simulink library "RflySimModelLab"  (R2022a)
settings: Solver=VariableStepAuto  StartTime=0.0  StopTime=10.0  RelTol=1e-3
values from neighbouring files (symbols this model uses):
  ESC = [ESC,ESCTmp]    [USV_init.m]
  motor = [motor,motorTmp]    [USV_init.m]
undefined symbols (not defined in the file or in its folder): LiftDrag
libraries: $bdroot x24, vrlib x3, aerolibasang x1, aerolibtransform2 x1
settings Model: Creator=dream  LastModifiedBy=dzl20201126
settings SolverCC: AlgebraicLoopSolver=TrustRegion
settings DataIOCC: ReturnWorkspaceOutputs=off
settings DebuggingCC: UnconnectedInputMsg=warning  UnconnectedOutputMsg=warning  UnconnectedLineMsg=warning  SFMachineParentedDataDiag=warning  ArithmeticOperatorsInVariantConditions=warning
settings SFSimCC: SimUseLocalCustomCode=off  CustomCodeUndefinedFunction=UseInterfaceOnly
settings RTWCC: RTWUseLocalCustomCode=off

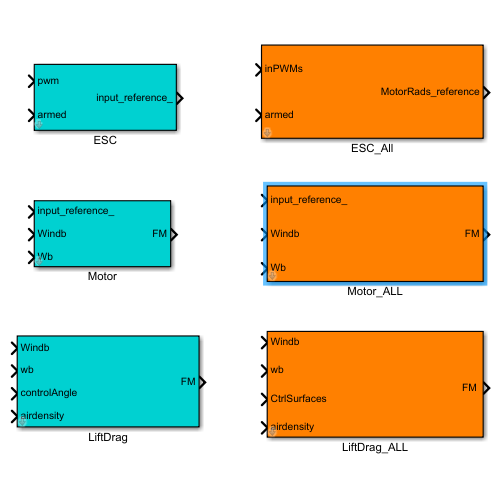
[thumbnail: Simulink's stored preview of the top-level diagram]
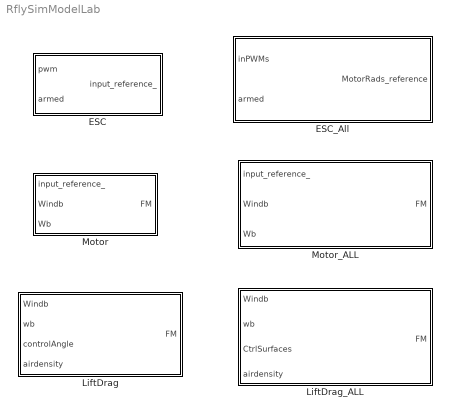
== system RflySimModelLab ==
  ESC : Subsystem  mask{MotorPara=ESC(1)}
      mask prompts: MotorPara "电机名"
  ESC_All : Subsystem  mask{ESCParam=ESC}
      mask prompts: ESCParam "电调参数"
  LiftDrag : Subsystem  mask{LiftDragParam=LiftDrag(1)}
      mask prompts: LiftDragParam "参数结构体"
  LiftDrag_ALL : Subsystem  mask{LiftDrag=LiftDrag}
      mask prompts: LiftDrag "部件参数结构体向量"
  Motor : Subsystem  mask{MotorPara=motor(1)}
      mask prompts: MotorPara "电机名"
  Motor_ALL : Subsystem  mask{MotorParam=motor}
      mask prompts: MotorParam "电机参数"

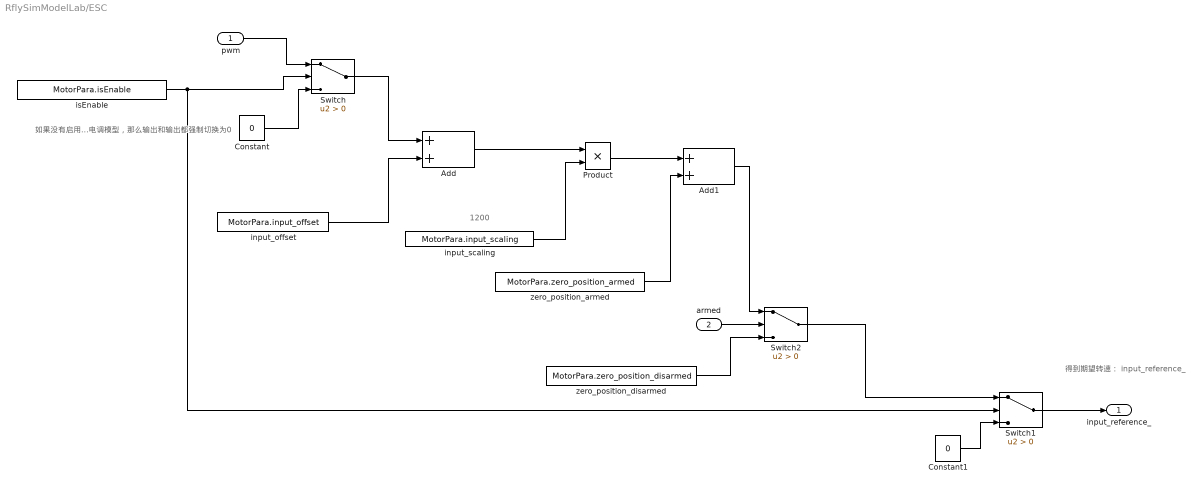
== system RflySimModelLab/ESC ==
  note: 如果没有启用电调模型，那么输出和输出都强制切换为0
  note: 1200
  note: 得到期望转速：
      | input_reference_
  pwm : Inport
  armed : Inport  Port=2
  Add : Sum
  Add1 : Sum
  Constant : Constant  Value=0
  Constant1 : Constant  Value=0
  Product : Product
  Switch : Switch  Criteria=u2 > Threshold  SaturateOnIntegerOverflow=off  InputSameDT=off
  Switch1 : Switch  Criteria=u2 > Threshold  SaturateOnIntegerOverflow=off  InputSameDT=off
  Switch2 : Switch  Criteria=u2 > Threshold  SaturateOnIntegerOverflow=off  InputSameDT=off
  input_offset : Constant  Value=MotorPara.input_offset
  input_scaling : Constant  Value=MotorPara.input_scaling
  isEnable : Constant  Value=MotorPara.isEnable
  zero_position_armed : Constant  Value=MotorPara.zero_position_armed
  zero_position_disarmed : Constant  Value=MotorPara.zero_position_disarmed
  input_reference_ : Outport  VectorParamsAs1DForOutWhenUnconnected=off
  wires:
  Product/1 -> Add1/1
  input_scaling/1 -> Product/2
  pwm/1 -> Switch/1
  Switch2/1 -> Switch1/1
  zero_position_armed/1 -> Add1/2
  input_offset/1 -> Add/2
  Add/1 -> Product/1
  isEnable/1 -> Switch/2, Switch1/2
  Constant/1 -> Switch/3
  Switch/1 -> Add/1
  Constant1/1 -> Switch1/3
  Switch1/1 -> input_reference_/1
  armed/1 -> Switch2/2
  Add1/1 -> Switch2/1
  zero_position_disarmed/1 -> Switch2/3

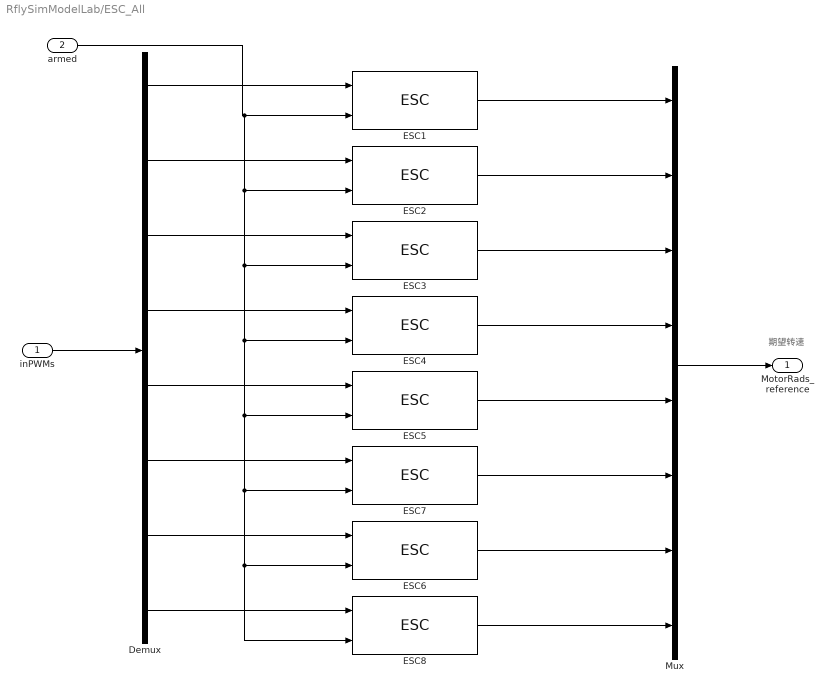
== system RflySimModelLab/ESC_All ==
  note: 期望转速
  inPWMs : Inport  PortDimensions=8
  armed : Inport  Port=2  PortDimensions=1
  Demux : Demux  Outputs=8
  ESC1 : $bdroot/ESC  MotorPara=ESCParam(1)
  ESC2 : $bdroot/ESC  MotorPara=ESCParam(2)
  ESC3 : $bdroot/ESC  MotorPara=ESCParam(3)
  ESC4 : $bdroot/ESC  MotorPara=ESCParam(4)
  ESC5 : $bdroot/ESC  MotorPara=ESCParam(5)
  ESC6 : $bdroot/ESC  MotorPara=ESCParam(7)
  ESC7 : $bdroot/ESC  MotorPara=ESCParam(6)
  ESC8 : $bdroot/ESC  MotorPara=ESCParam(8)
  Mux : Mux  Inputs=8
  MotorRads_reference : Outport  VectorParamsAs1DForOutWhenUnconnected=off
  wires:
  ESC2/1 -> Mux/2
  ESC1/1 -> Mux/1
  Demux/2 -> ESC2/1
  Demux/1 -> ESC1/1
  Demux/3 -> ESC3/1
  ESC3/1 -> Mux/3
  Demux/4 -> ESC4/1
  ESC4/1 -> Mux/4
  Demux/5 -> ESC5/1
  ESC5/1 -> Mux/5
  Demux/6 -> ESC7/1
  ESC7/1 -> Mux/6
  Demux/7 -> ESC6/1
  ESC6/1 -> Mux/7
  Demux/8 -> ESC8/1
  ESC8/1 -> Mux/8
  Mux/1 -> MotorRads_reference/1
  inPWMs/1 -> Demux/1
  armed/1 -> ESC8/2, ESC6/2, ESC7/2, ESC5/2, ESC4/2, ESC3/2, ESC2/2, ESC1/2

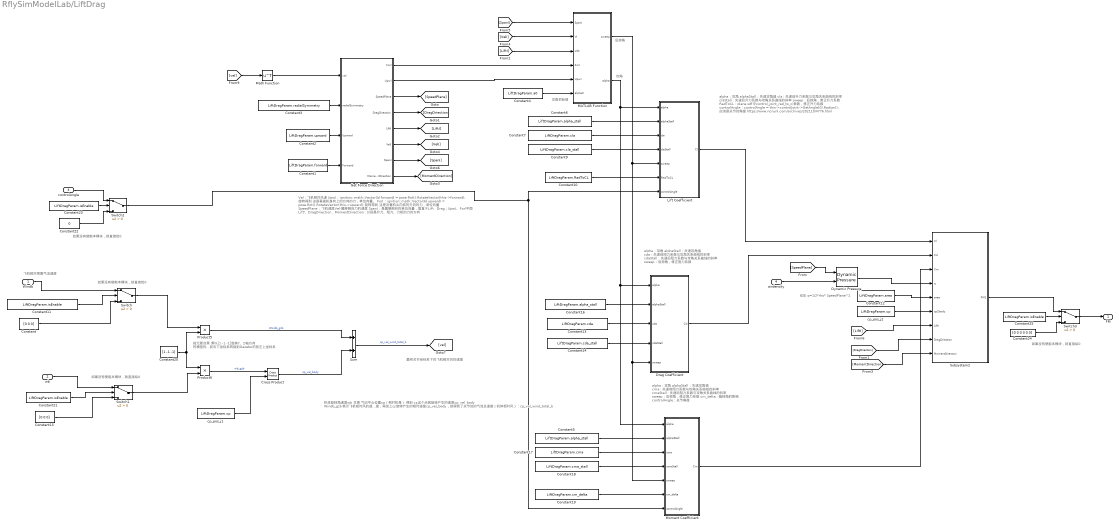
== system RflySimModelLab/LiftDrag ==
  note: alpha：攻角
      | alphaStall：失速攻角值
      | cla：失速前升力系数与攻角关系曲线的斜率
      | claStall：失速后升力系数与攻角关系曲线的斜率
      | sweep：后掠角，修正升力系数
      | RadToCL：plane sdf中control_joint_rad_to_cl参数，修正升力系数
      | controlAngle：controlAngle = this->controlJoint->GetAngle(0).Radian();
      | 应该是关节的角度
      |
      | https://www.ncnynl.com/archives/202110/4776.html
  note: 动压 q=1/2*rho* SpeedPlane^2
  note: 按元素点乘
      | 乘以[1 -1 -1]变换Y、Z轴方向
      | 将模型的前右下坐标系转换到Gazebo的前左上坐标系
  note: 攻角初始值
  note: 机体旋转角速度wb 叉乘 气动中心位置cp（相对机身） 得到 cp这个点因旋转产生的速度cp_vel_body
      |
      | Windb_gzb表示飞机相对风的速度，再加上cp旋转产生的相对速度cp_vel_body，就得到了关节处的气流总速度（机体相对风）：cp_vel_wind_total_b
  note: 如果没有使能本模块，就直接给0
  note: 飞机相对周围气流速度
  note: alpha：攻角
      | alphaStall：失速攻角值
      | cma：失速前阻力系数与攻角关系曲线的斜率
      | cmaStall：失速后阻力系数与攻角关系曲线的斜率
      | sweep：后掠角，修正阻力系数
      | cm_delta：偏转角的影响
      | controlAngle：关节角度
  note: 如果没有使能本模块，就直接给0
  note: 攻角
  note: 如果没有使能本模块，就直接给0
  note: 后掠角
  note: 如果没有使能本模块，就直接给0
  note: 最终关节坐标系下的飞机相对风的速度
  note: Vel：飞机相对风速
      | UpwI：ignition::math::Vector3d forwardI = pose.Rot().RotateVector(this->forward); 旋转得到
      | 	    这是垂直机身向上的方向的力，单位向量。
      | ForI：ignition::math::Vector3d upwardI = pose.Rot().RotateVector(this->upward);旋转得到
      | 	    这是沿着机头向前的方向的力，单位向量
      |
      | SpeedPlane：飞机速度Vel-翼展侧向力的速度
      | SpanI：是翼展侧向的单位向量，垂直于Lift、Drag；UpwI、ForI平面
      | LiftI、DragDriection、MomentDirection：分别是升力、阻力、力矩的力的方向
  note: alpha：攻角
      | alphaStall：失速攻角值
      | cda：失速前阻力系数与攻角关系曲线的斜率
      | cdaStall：失速后阻力系数与攻角关系曲线的斜率
      | sweep：后掠角，修正阻力系数
  Windb : Inport
  wb : Inport  Port=2
  controlAngle : Inport  Port=3
  airdensity : Inport  Port=4
  Constant : Constant  Value=[0 0 0]  VectorParams1D=off
  Constant1 : Constant  Value=LiftDragParam.forward  VectorParams1D=off
  Constant10 : Constant  Value=LiftDragParam.RadToCL
  Constant{11,21,23,25} (4 alike) : Constant  Value=LiftDragParam.isEnable
  Constant12 : Constant  Value=LiftDragParam.area
  Constant13 : Constant  Value=LiftDragParam.cda
  Constant14 : Constant  Value=LiftDragParam.cda_stall
  Constant15 : Constant  Value=[0 0 0]  VectorParams1D=off
  Constant16 : Constant  Value=LiftDragParam.alpha_stall
  Constant17 : Constant  Value=LiftDragParam.cma
  Constant18 : Constant  Value=LiftDragParam.cma_stall
  Constant19 : Constant  Value=LiftDragParam.cm_delta
  Constant2 : Constant  Value=LiftDragParam.upward  VectorParams1D=off
  Constant20 : Constant  Value=[1 -1 -1]  VectorParams1D=off
  Constant22 : Constant  Value=0
  Constant24 : Constant  Value=[0 0 0 0 0 0]
  Constant3 : Constant  Value=LiftDragParam.radialSymmetry
  Constant4 : Constant  Value=LiftDragParam.a0
  Constant5 : Constant  Value=LiftDragParam.alpha_stall
  Constant6 : Constant  Value=LiftDragParam.alpha_stall
  Constant7 : Constant  Value=LiftDragParam.cla
  Constant9 : Constant  Value=LiftDragParam.cla_stall
  Cross Product : vrlib/Utilities/Cross Product
  Drag Coefficient : MATLAB Function  TreatAsAtomicUnit=on
  Dynamic Pressure : aerolibasang/Dynamic Pressure
  Get Force Direction : MATLAB Function  Description=dddddd  TreatAsAtomicUnit=on
  Lift Coefficient : MATLAB Function  TreatAsAtomicUnit=on
  MATLAB Function : MATLAB Function  TreatAsAtomicUnit=on
  Math Function : Math  Operator=transpose  SignedPower=on
  Moment Coefficient : MATLAB Function  TreatAsAtomicUnit=on
  Product5 : Product
  Product6 : Product
  Subsystem2 : Subsystem
  Sum : Sum
  Switch{,1..3} (4 alike) : Switch  Criteria=u2 > Threshold  SaturateOnIntegerOverflow=off  InputSameDT=off
  cp_pos_j1 : Constant  Value=LiftDragParam.cp
  cp_pos_j2 : Constant  Value=LiftDragParam.cp
  FM : Outport  VectorParamsAs1DForOutWhenUnconnected=off
  wires:
  Constant16/1 -> Drag Coefficient/2(alphaStall)
  Windb/1 -> Switch/1
  Sum/1 -> [vel]  "cp_vel_wind_total_b"
  Constant17/1 -> Moment Coefficient/3(cma)
  Constant7/1 -> Lift Coefficient/3(cla)
  Get Force Direction/3(SpeedPlane) -> [SpeedPlane]
  Get Force Direction/6(VelI) -> [VelI]
  Constant19/1 -> Moment Coefficient/6(cm_delta)
  Dynamic Pressure/1 -> Subsystem2/4(q)
  Get Force Direction/7(SpanI) -> [SpanI]
  Constant6/1 -> Lift Coefficient/2(alphaStall)
  Constant13/1 -> Drag Coefficient/3(cda)
  Constant14/1 -> Drag Coefficient/4(cdaStall)
  Constant9/1 -> Lift Coefficient/4(claStall)
  Constant20/1 -> Product5/2, Product6/1
  Constant1/1 -> Get Force Direction/4(Forward)
  [VelI] -> MATLAB Function/2(VI)
  MATLAB Function/1(sweep) -> Lift Coefficient/5(sweep), Drag Coefficient/5(sweep), Moment Coefficient/5(sweep)
  airdensity/1 -> Dynamic Pressure/2
  MATLAB Function/2(alpha) -> Drag Coefficient/1(alpha), Moment Coefficient/1(alpha), Lift Coefficient/1(alpha)
  Get Force Direction/4(DragDirection) -> [DragDriection]
  Constant3/1 -> Get Force Direction/2(radialSymmetry)
  cp_pos_j1/1 -> Cross Product/2
  Constant10/1 -> Lift Coefficient/6(RadToCL)
  Get Force Direction/5(LiftI) -> [LiftI]
  Constant25/1 -> Switch3/2
  Constant5/1 -> Moment Coefficient/2(alphaStall)
  [SpeedPlane] -> Dynamic Pressure/1
  Lift Coefficient/1(Cl) -> Subsystem2/1(Cl)
  Constant4/1 -> MATLAB Function/6(alpha0)
  Moment Coefficient/1(Cm) -> Subsystem2/3(Cm)
  [LiftI] -> Subsystem2/7(LiftI)
  [vel] -> Math Function/1
  cp_pos_j2/1 -> Subsystem2/6(cp2body)
  Cross Product/1 -> Sum/2  "cp_vel_body"
  Get Force Direction/2(UpwI) -> MATLAB Function/5(UpwI)
  [SpanI] -> MATLAB Function/1(SpanI)
  controlAngle/1 -> Switch2/1
  Switch/1 -> Product5/1
  Constant18/1 -> Moment Coefficient/4(cmaStall)
  Get Force Direction/1(ForI) -> MATLAB Function/4(ForI)
  Constant11/1 -> Switch/2
  Get Force Direction/8(MomentDirection) -> [MomentDirection]
  Switch1/1 -> Product6/2
  Product5/1 -> Sum/1  "Windb_gzb"
  Switch2/1 -> Lift Coefficient/7(controlAngle), Moment Coefficient/7(controlAngle)
  Product6/1 -> Cross Product/1  "wb_gzb"
  Constant/1 -> Switch/3
  [MomentDirection] -> Subsystem2/9(MomentDirection)
  Drag Coefficient/1(Cd) -> Subsystem2/2(Cd)
  [DragDriection] -> Subsystem2/8(DragDriection)
  Constant12/1 -> Subsystem2/5(area)
  Constant23/1 -> Switch2/2
  Constant2/1 -> Get Force Direction/3(Upward)
  Subsystem2/1(FM1) -> Switch3/1
  [LiftI] -> MATLAB Function/3(LiftI)
  Constant15/1 -> Switch1/3
  Constant21/1 -> Switch1/2
  Switch3/1 -> FM/1
  wb/1 -> Switch1/1
  Constant24/1 -> Switch3/3
  Math Function/1 -> Get Force Direction/1(vel)
  Constant22/1 -> Switch2/3

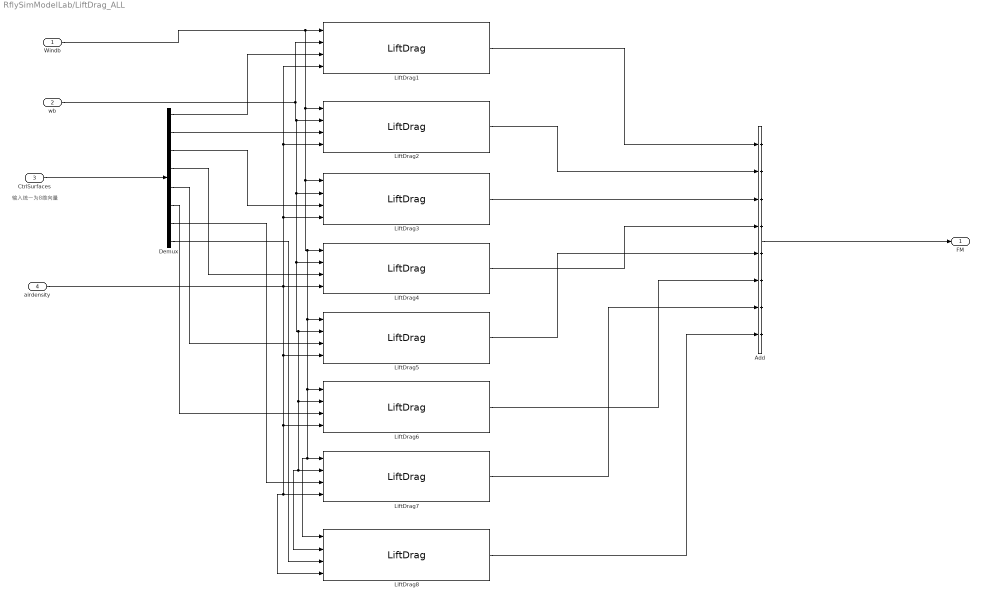
== system RflySimModelLab/LiftDrag_ALL ==
  note: 输入统一为8维向量
  Windb : Inport
  wb : Inport  Port=2
  CtrlSurfaces : Inport  Port=3  PortDimensions=8
  airdensity : Inport  Port=4
  Add : Sum  Inputs=++++++++
  Demux : Demux  Outputs=8
  LiftDrag1 : $bdroot/LiftDrag  LiftDragParam=LiftDrag(1)
  LiftDrag2 : $bdroot/LiftDrag  LiftDragParam=LiftDrag(2)
  LiftDrag3 : $bdroot/LiftDrag  LiftDragParam=LiftDrag(3)
  LiftDrag4 : $bdroot/LiftDrag  LiftDragParam=LiftDrag(4)
  LiftDrag5 : $bdroot/LiftDrag  LiftDragParam=LiftDrag(5)
  LiftDrag6 : $bdroot/LiftDrag  LiftDragParam=LiftDrag(6)
  LiftDrag7 : $bdroot/LiftDrag  LiftDragParam=LiftDrag(7)
  LiftDrag8 : $bdroot/LiftDrag  LiftDragParam=LiftDrag(8)
  "FM " : Outport
  wires:
  Windb/1 -> LiftDrag1/1, LiftDrag2/1, LiftDrag3/1, LiftDrag4/1, LiftDrag5/1, LiftDrag6/1, LiftDrag8/1, LiftDrag7/1
  wb/1 -> LiftDrag1/2, LiftDrag2/2, LiftDrag3/2, LiftDrag4/2, LiftDrag5/2, LiftDrag6/2, LiftDrag8/2, LiftDrag7/2
  Demux/2 -> LiftDrag2/3
  LiftDrag6/1 -> Add/6
  LiftDrag3/1 -> Add/3
  Demux/3 -> LiftDrag3/3
  Demux/4 -> LiftDrag4/3
  LiftDrag5/1 -> Add/5
  Demux/7 -> LiftDrag7/3
  Demux/5 -> LiftDrag5/3
  Demux/1 -> LiftDrag1/3
  airdensity/1 -> LiftDrag3/4, LiftDrag2/4, LiftDrag1/4, LiftDrag4/4, LiftDrag5/4, LiftDrag6/4, LiftDrag8/4, LiftDrag7/4
  Demux/6 -> LiftDrag6/3
  LiftDrag7/1 -> Add/7
  CtrlSurfaces/1 -> Demux/1
  Add/1 -> "FM "/1
  LiftDrag8/1 -> Add/8
  Demux/8 -> LiftDrag8/3
  LiftDrag2/1 -> Add/2
  LiftDrag4/1 -> Add/4
  LiftDrag1/1 -> Add/1

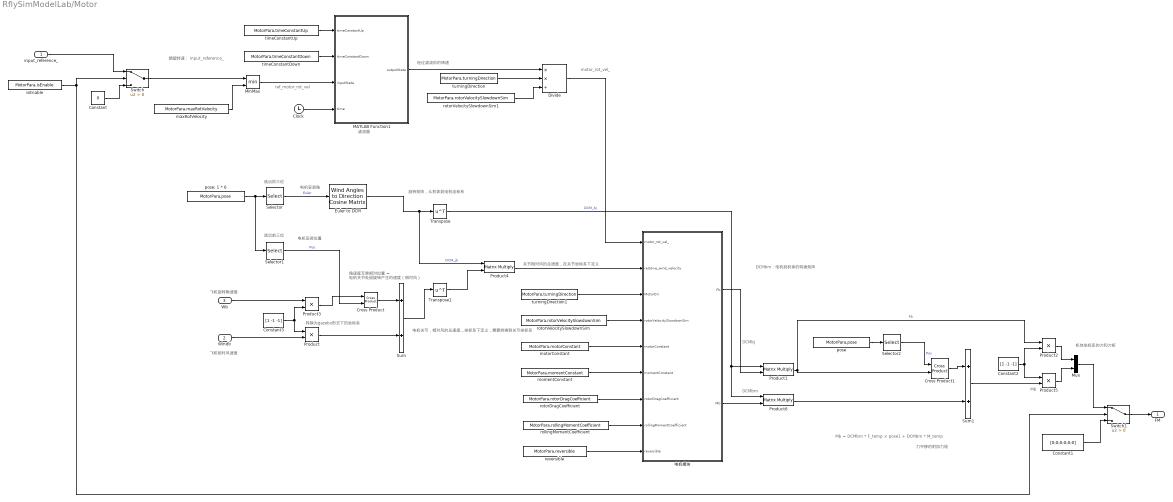
== system RflySimModelLab/Motor ==
  note: 关节相对风的总速度，在关节坐标系下定义
  note: 电机关节，相对风的总速度，在机体坐标系下定义，需要转换到关节坐标系
  note: 角速度叉乘相对位置 = 电机关节处因旋转产生的速度（相对风）
  note: 飞机旋转角速度
  note: 飞机相对风速度
  note: 电机安装位置
  note: 电机安装角
  note: 旋转矩阵，从机体到电机坐标系
  note: 选出后三位
  note: motor_rot_vel_
  note: 转换为gazebo形式下的坐标系
  note: 机体坐标系的力和力矩
  note: 力平移的附加力矩
  note: Mb
  note: DCMbm
  note: DCMbm：电机到机体的转换矩阵
  note: Mb = DCMbm * F_temp × pose1 + DCMbm * M_temp
  note: DCMbj
  note: ref_motor_rot_vel
  note: 经过滤波后的转速
  note: 滤波器
  note: 期望转速：
      | input_reference_
  note: 选出前三位
  input_reference_ : Inport
  Windb : Inport  Port=2
  Wb : Inport  Port=3
  Clock : Clock
  Constant : Constant  Value=0
  Constant1 : Constant  Value=[0;0;0;0;0;0]
  Constant2 : Constant  Value=[1 -1 -1]
  Constant3 : Constant  Value=[1 -1 -1]
  Cross Product : vrlib/Utilities/Cross Product
  Cross Product1 : vrlib/Utilities/Cross Product
  Divide : Product  Inputs=**/
  Euler to DCM : aerolibtransform2/Wind Angles to  Direction Cosine Matrix
      settings: SourceProductBaseCode=AE
  MATLAB Function1 : MATLAB Function  TreatAsAtomicUnit=on
  MinMax : MinMax  Inputs=2
  Mux : Mux  Inputs=2
  Product{,2..3,5} (4 alike) : Product
  Product1 : Product  Multiplication=Matrix(*)
  Product4 : Product  Multiplication=Matrix(*)
  Product6 : Product  Multiplication=Matrix(*)
  Selector : Selector  InputPortWidth=6  IndexOptions=Starting index (dialog)  Indices=[4]  OutputSizes=3
  Selector1 : Selector  InputPortWidth=6  IndexOptions=Starting index (dialog)  Indices=[1]  OutputSizes=3
  Selector2 : Selector  InputPortWidth=6  IndexOptions=Starting index (dialog)  Indices=[1]  OutputSizes=3
  Sum : Sum
  Sum1 : Sum
  Switch : Switch  Criteria=u2 > Threshold  SaturateOnIntegerOverflow=off  InputSameDT=off
  Switch1 : Switch  Criteria=u2 > Threshold  SaturateOnIntegerOverflow=off  InputSameDT=off
  Transpose : Math  Operator=transpose  SignedPower=on
  Transpose1 : Math  Operator=transpose  SignedPower=on
  isEnable : Constant  Value=MotorPara.isEnable
  maxRotVelocity : Constant  Value=MotorPara.maxRotVelocity
  momentConstant : Constant  Value=MotorPara.momentConstant
  motorConstant : Constant  Value=MotorPara.motorConstant
  pose : Constant  Value=MotorPara.pose
  pose: 1 * 6 : Constant  Value=MotorPara.pose
  reversible : Constant  Value=MotorPara.reversible
  rollingMomentCoefficient : Constant  Value=MotorPara.rollingMomentCoefficient
  rotorDragCoefficient : Constant  Value=MotorPara.rotorDragCoefficient
  rotorVelocitySlowdownSim : Constant  Value=MotorPara.rotorVelocitySlowdownSim
  rotorVelocitySlowdownSim1 : Constant  Value=MotorPara.rotorVelocitySlowdownSim
  timeConstantDown : Constant  Value=MotorPara.timeConstantDown
  timeConstantUp : Constant  Value=MotorPara.timeConstantUp
  turningDirection : Constant  Value=MotorPara.turningDirection
  turningDirection1 : Constant  Value=MotorPara.turningDirection
  电机模块 : MATLAB Function  TreatAsAtomicUnit=on
  FM : Outport
  wires:
  rotorVelocitySlowdownSim/1 -> 电机模块/4(rotorVelocitySlowdownSim)
  rollingMomentCoefficient/1 -> 电机模块/8(rollingMomentCoefficient)
  motorConstant/1 -> 电机模块/5(motorConstant)
  momentConstant/1 -> 电机模块/6(momentConstant)
  rotorDragCoefficient/1 -> 电机模块/7(rotorDragCoefficient)
  turningDirection1/1 -> 电机模块/3(MotorDir)
  Product4/1 -> 电机模块/2(relative_wind_velocity)
  Product2/1 -> Mux/1
  Product5/1 -> Mux/2
  Constant2/1 -> Product5/1, Product2/2
  Euler to DCM/1 -> Product4/1, Transpose/1  "DCM_jb"
  Constant3/1 -> Product3/2, Product/1
  Wb/1 -> Product3/1
  Product3/1 -> Cross Product/1
  Cross Product/1 -> Sum/1
  Product/1 -> Sum/2
  Sum/1 -> Transpose1/1
  电机模块/1(Fb) -> Product1/2
  Product1/1 -> Cross Product1/2, Product2/1  "Fb"
  Cross Product1/1 -> Sum1/1
  Sum1/1 -> Product5/2
  电机模块/2(Mb) -> Product6/2
  Product6/1 -> Sum1/2
  Mux/1 -> Switch1/1
  Transpose1/1 -> Product4/2
  timeConstantDown/1 -> MATLAB Function1/2(timeConstantDown)
  timeConstantUp/1 -> MATLAB Function1/1(timeConstantUp)
  Clock/1 -> MATLAB Function1/4(time)
  Switch/1 -> MinMax/1
  maxRotVelocity/1 -> MinMax/2
  MinMax/1 -> MATLAB Function1/3(inputState)
  MATLAB Function1/1(outputState) -> Divide/1
  rotorVelocitySlowdownSim1/1 -> Divide/3
  turningDirection/1 -> Divide/2
  pose: 1 * 6/1 -> Selector1/1, Selector/1
  Selector/1 -> Euler to DCM/1  "Euler"
  Selector1/1 -> Cross Product/2  "Pos"
  pose/1 -> Selector2/1
  Selector2/1 -> Cross Product1/1  "Pos"
  reversible/1 -> 电机模块/9(reversible)
  Divide/1 -> 电机模块/1(motor_rot_vel_)
  isEnable/1 -> Switch/2, Switch1/2
  Constant/1 -> Switch/3
  input_reference_/1 -> Switch/1
  Constant1/1 -> Switch1/3
  Switch1/1 -> FM/1
  Transpose/1 -> Product6/1, Product1/1  "DCM_bj"
  Windb/1 -> Product/2

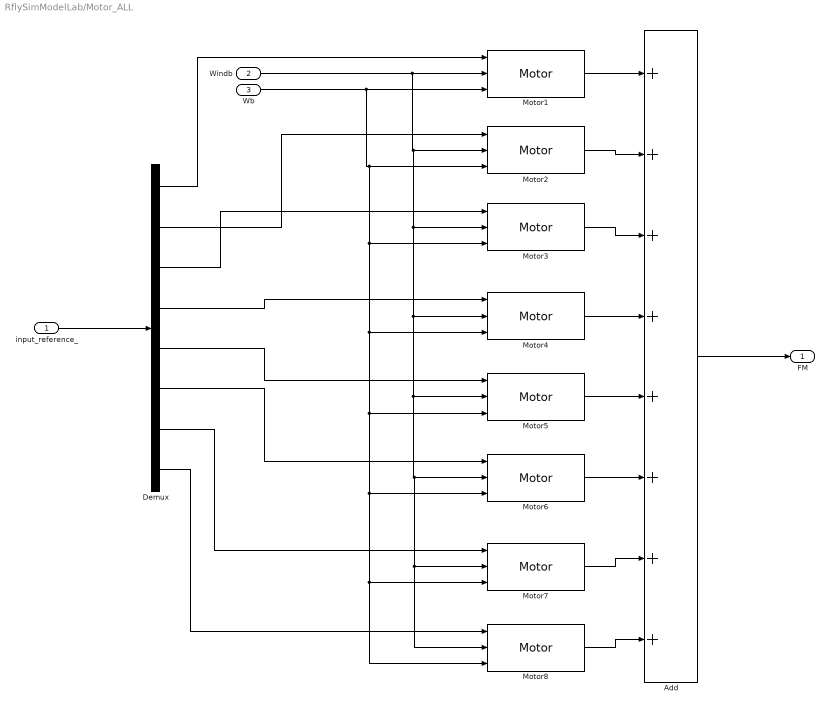
== system RflySimModelLab/Motor_ALL ==
  input_reference_ : Inport
  Windb : Inport  Port=2
  Wb : Inport  Port=3
  Add : Sum  Inputs=++++++++
  Demux : Demux  Outputs=8
  Motor1 : $bdroot/Motor  MotorPara=MotorParam(1)
  Motor2 : $bdroot/Motor  MotorPara=MotorParam(2)
  Motor3 : $bdroot/Motor  MotorPara=MotorParam(3)
  Motor4 : $bdroot/Motor  MotorPara=MotorParam(4)
  Motor5 : $bdroot/Motor  MotorPara=MotorParam(5)
  Motor6 : $bdroot/Motor  MotorPara=MotorParam(6)
  Motor7 : $bdroot/Motor  MotorPara=MotorParam(7)
  Motor8 : $bdroot/Motor  MotorPara=MotorParam(8)
  FM : Outport
  wires:
  Wb/1 -> Motor5/3, Motor7/3, Motor8/3, Motor6/3, Motor4/3, Motor3/3, Motor2/3, Motor1/3
  Windb/1 -> Motor8/2, Motor7/2, Motor6/2, Motor5/2, Motor4/2, Motor3/2, Motor2/2, Motor1/2
  Demux/1 -> Motor1/1
  input_reference_/1 -> Demux/1
  Demux/2 -> Motor2/1
  Demux/3 -> Motor3/1
  Demux/4 -> Motor4/1
  Demux/5 -> Motor5/1
  Demux/6 -> Motor6/1
  Demux/7 -> Motor7/1
  Demux/8 -> Motor8/1
  Motor1/1 -> Add/1
  Motor2/1 -> Add/2
  Motor3/1 -> Add/3
  Motor4/1 -> Add/4
  Motor5/1 -> Add/5
  Motor6/1 -> Add/6
  Motor7/1 -> Add/7
  Motor8/1 -> Add/8
  Add/1 -> FM/1

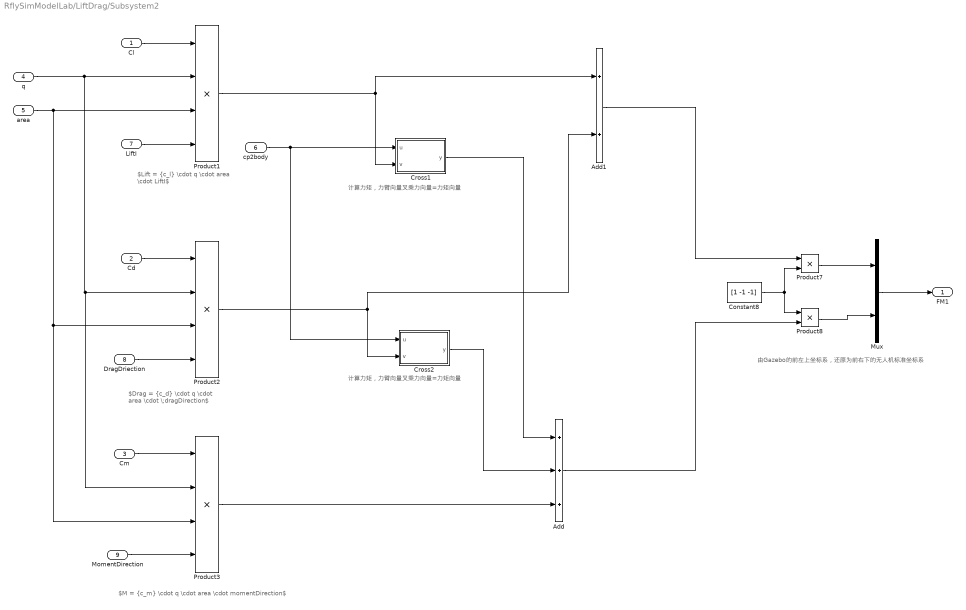
== system RflySimModelLab/LiftDrag/Subsystem2 ==
  note: $Drag = {c_d} \cdot q \cdot area \cdot \;dragDirection$
  note: 计算力矩，力臂向量叉乘力向量=力矩向量
  note: $M = {c_m} \cdot q \cdot area \cdot momentDirection$
  note: 计算力矩，力臂向量叉乘力向量=力矩向量
  note: 由Gazebo的前左上坐标系，还原为前右下的无人机标准坐标系
  note: $Lift = {c_l} \cdot q \cdot area \cdot LiftI$
  Cl : Inport
  Cd : Inport  Port=2
  Cm : Inport  Port=3
  q : Inport  Port=4
  area : Inport  Port=5
  cp2body : Inport  Port=6
  LiftI : Inport  Port=7
  DragDriection : Inport  Port=8
  MomentDirection : Inport  Port=9
  Add : Sum  Inputs=+++
  Add1 : Sum
  Constant8 : Constant  Value=[1 -1 -1]
  Cross1 : MATLAB Function  TreatAsAtomicUnit=on
  Cross2 : MATLAB Function  TreatAsAtomicUnit=on
  Mux : Mux  Inputs=2
  Product1 : Product  Inputs=4
  Product2 : Product  Inputs=4
  Product3 : Product  Inputs=4
  Product7 : Product
  Product8 : Product
  FM1 : Outport
  wires:
  Product2/1 -> Add1/2, Cross2/2(v)
  Add1/1 -> Product7/1
  Cm/1 -> Product3/1
  LiftI/1 -> Product1/4
  Product3/1 -> Add/3
  Cross2/1(y) -> Add/2
  Cl/1 -> Product1/1
  Cross1/1(y) -> Add/1
  MomentDirection/1 -> Product3/4
  Product1/1 -> Add1/1, Cross1/2(v)
  Cd/1 -> Product2/1
  Product8/1 -> Mux/2
  Constant8/1 -> Product8/1, Product7/2
  Mux/1 -> FM1/1
  Add/1 -> Product8/2
  Product7/1 -> Mux/1
  cp2body/1 -> Cross2/1(u), Cross1/1(u)
  area/1 -> Product3/3, Product2/3, Product1/3
  DragDriection/1 -> Product2/4
  q/1 -> Product3/2, Product2/2, Product1/2

== matlab function RflySimModelLab/LiftDrag/Subsystem2/Cross1 ==
  data: u input; y output; v input
function y = fcn(u, v)
    y = cross(u, v);
end

== matlab function RflySimModelLab/LiftDrag/Subsystem2/Cross2 ==
  data: u input; y output; v input
function y = fcn(u, v)
    y = cross(u, v);
end

== matlab function RflySimModelLab/Motor/电机模块 ==
  data: motor_rot_vel_ input; relative_wind_velocity input; MotorDir input; rotorVelocitySlowdownSim input; motorConstant input; momentConstant input; rotorDragCoefficient input; Fb output; Mb output; rollingMomentCoefficient input; reversible input
function [Fb,Mb] = fcn(motor_rot_vel_,relative_wind_velocity,MotorDir,...
    rotorVelocitySlowdownSim,motorConstant,momentConstant,rotorDragCoefficient,...
   rollingMomentCoefficient,reversible)
% This is control effectiveness model, where Fb is the force produced by motors, Mb is
% the moment produced by motors, and Fd is the resistance produced by the air.
% The gyroscopic torque is not considered here.

% -1: anticlockwise, 1: clockwise 

Mb = [0;0;0];
Fb = [0;0;0];

propdir = MotorDir;
real_motor_velocity = motor_rot_vel_ * rotorVelocitySlowdownSim;

% 相对风速分量
velocity_perpendicular_to_rotor_axis = [relative_wind_velocity(1);relative_wind_velocity(2);0];
velocity_parallel_to_rotor_axis = [0;0;relative_wind_velocity(3)];
vel = abs(relative_wind_velocity(3));
scalar = 1 - vel/25.0;
if scalar<0
    scalar = 0;
elseif scalar>1
        scalar = 0;
end
% 推力 % Fm应用到模型上之前还需要根据与水流/风速的相对速度进行缩放，scale：0-1
force = real_motor_velocity * abs(real_motor_velocity) * motorConstant;
if reversible==0          % 表示电机不能有负推力
    force = abs(force);
end
Fm1 = [0;0;force * scalar];
%  旋翼的气动阻力
% relative_wind_velocity = body_velocity - wind_vel_;
% velocity_perpendicular_to_rotor_axis = relative_wind_velocity - (relative_wind_velocity.*(joint_axis)) .* joint_axis;
Fm2 = -abs(real_motor_velocity) * rotorDragCoefficient * velocity_perpendicular_to_rotor_axis;
Fb = Fm1 + Fm2;

% 用于偏航的空气阻力矩  Mt1     
Mt1 = [0;0;-propdir*force*momentConstant];    % gazebo中ccw对应1，而这里对应-1，所以propdir前没负号
% 滚动力矩Mt2
Mt2 = -abs(real_motor_velocity) * rollingMomentCoefficient * velocity_perpendicular_to_rotor_axis;
Mb = Mt1 + Mt2;

end

== matlab function RflySimModelLab/Motor/MATLAB Function1 ==
  settings: updateMethod=DISCRETE
  data: timeConstantUp input; outputState output; timeConstantDown input; inputState input; time input
function outputState = fcn(timeConstantUp, timeConstantDown, inputState, time)
persistent previousState;
if isempty(previousState)
    previousState=0;
end

persistent lastTime;
if isempty(lastTime)
    lastTime=0;
end

samplingTime=time-lastTime;
if samplingTime<=0
    samplingTime=0.01;
end

if inputState > previousState
    alphaUp = exp(-samplingTime/timeConstantUp);
    outputState = alphaUp*previousState + (1-alphaUp)*inputState;
else
    alphaDown = exp(- samplingTime / timeConstantDown);
    outputState = alphaDown*previousState + (1-alphaDown)*inputState;
end

previousState=inputState;
lastTime=time;

== matlab function RflySimModelLab/LiftDrag/Drag Coefficient ==
  data: alpha input; Cd output; alphaStall input; cda input; cdaStall input; sweep input
function Cd= fcn(alpha, alphaStall, cda, cdaStall, sweep)
    if alpha>alphaStall
        Cd = (cda*alphaStall + cdaStall*(alpha-alphaStall))*cos(sweep);
    elseif alpha< -alphaStall
        Cd = (-cda*alphaStall + cdaStall*(alpha+alphaStall))*cos(sweep);
    else
        Cd = cda*alpha*cos(sweep);
    end
    
    Cd = abs(Cd);

== matlab function RflySimModelLab/LiftDrag/Get Force Direction ==
  data: ForI output; UpwI output; vel input; radialSymmetry input; SpeedPlane output; Upward input; DragDirection output; LiftI output; VelI output; SpanI output; MomentDirection output; Forward input
function [ForI, UpwI, SpeedPlane, DragDirection, LiftI, VelI, SpanI, MomentDirection] = fcn(vel, radialSymmetry, Upward, Forward)
    if norm(vel)>1e-6
        VelI = vel/norm(vel);                   %模块输入vel是部件坐标系下相对风速
    else
        VelI = zeros(3,1);
    end
    ForI = Forward;
    if radialSymmetry
        tmp = cross(ForI, VelI);
        UpwI = cross(ForI, tmp);
    else
        UpwI = Upward;
    end

    SpanI = cross(ForI, UpwI);
    if norm(SpanI)>1e-6
        SpanI = SpanI/norm(SpanI);
    else
        SpanI = zeros(3,1);
    end

    velPlane = vel - dot(vel, SpanI)*SpanI;
    DragDirection = - velPlane;
    if norm(DragDirection)>1e-6
        DragDirection = DragDirection/norm(DragDirection);
    else
        DragDirection = zeros(3,1);
    end
    
    
    tmp = cross(SpanI, velPlane);
    if norm(tmp)>1e-6
        LiftI = tmp/norm(tmp);
    else
        LiftI = zeros(3,1);
    end
 
    MomentDirection = SpanI;
    SpeedPlane = velPlane;

== matlab function RflySimModelLab/LiftDrag/Lift Coefficient ==
  data: alpha input; Cl output; alphaStall input; cla input; claStall input; sweep input; RadToCL input; controlAngle input
function Cl= fcn(alpha, alphaStall, cla, claStall, sweep, RadToCL, controlAngle)
    if alpha>alphaStall
        cl = (cla*alphaStall + claStall*(alpha-alphaStall))*cos(sweep);
        cl = max(0.0, cl);
    elseif alpha< -alphaStall
        cl = (-cla*alphaStall + claStall*(alpha+alphaStall))*cos(sweep);
        cl = min(0.0, cl);
    else
        cl = cla*alpha*cos(sweep);
    end
    
    Cl = cl + RadToCL*controlAngle;

== matlab function RflySimModelLab/LiftDrag/MATLAB Function ==
  data: SpanI input; sweep output; VI input; LiftI input; ForI input; UpwI input; alpha output; alpha0 input
function [sweep, alpha] = fcn(SpanI, VI, LiftI, ForI, UpwI, alpha0)
   sin_sweep =  dot(SpanI, VI);
   if sin_sweep > 1
       sin_sweep = 1;
   elseif sin_sweep < -1
       sin_sweep = -1;
   end
   sweep_0 = asin(sin_sweep);
   
   if abs(sweep_0) > pi/2
       if sweep_0 >0
           sweep_0 = sweep_0 - pi;
       else
           sweep_0 = sweep_0 + pi;
       end
   end
   
   cosalpha = dot(LiftI, UpwI);
   if cosalpha > 1
       cosalpha = 1;
   elseif cosalpha < -1
       cosalpha = -1;
   end
       
   if dot(LiftI, ForI) >=0
       alp =alpha0 + acos(cosalpha);
   else
       alp =alpha0 - acos(cosalpha);
   end
       
   if abs(alp) > pi/2
       if alp >0
           alp = alp - pi;
       else
           alp = alp + pi;
       end
   end
    
   
sweep = sweep_0;
alpha = alp;

== matlab function RflySimModelLab/LiftDrag/Moment Coefficient ==
  data: alpha input; Cm output; alphaStall input; cma input; cmaStall input; sweep input; cm_delta input; controlAngle input
function Cm= fcn(alpha, alphaStall, cma, cmaStall, sweep, cm_delta, controlAngle)
    if alpha>alphaStall
        Cm = (cma*alphaStall + cmaStall*(alpha-alphaStall))*cos(sweep);
        Cm = max(0.0, Cm);
    elseif alpha< -alphaStall
        Cm = (-cma*alphaStall + cmaStall*(alpha+alphaStall))*cos(sweep);
        Cm = min(0.0, Cm);
    else
        Cm = cma*alpha*cos(sweep);
    end
    
    Cm = Cm + cm_delta*controlAngle;
